simulink model "Vibro_Simulink Model"  (R2023a)
settings: Solver=VariableStepAuto  StartTime=0.0  StopTime=inf  RelTol=1e-3
undefined symbols (not defined in the file): f
libraries: instrumentlib x1
settings Model: Creator=Krishna Praveen  LastModifiedBy=Krishna Praveen

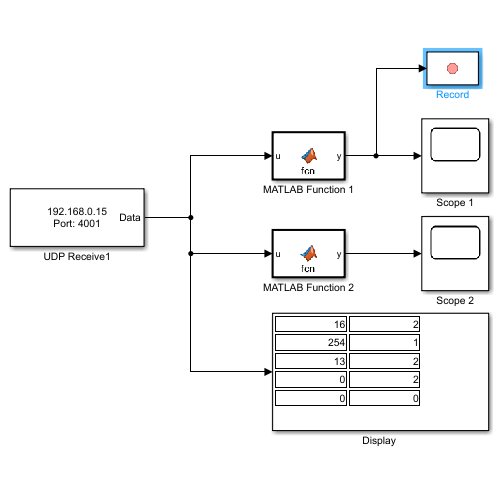
[thumbnail: Simulink's stored preview of the top-level diagram]
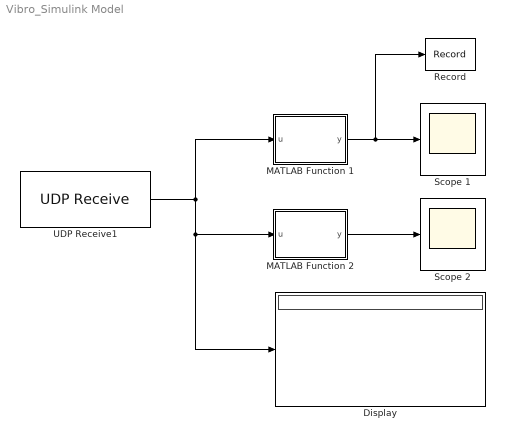
== system Vibro_Simulink Model ==
  "Display " : Display
  MATLAB Function 1 : MATLAB Function  TreatAsAtomicUnit=on
  MATLAB Function 2 : MATLAB Function  TreatAsAtomicUnit=on
  Record : Record  FileSettingsInternal="{\"entries\":[{\"content\":{\"excelSettings\":{\"content\":{},\"type\":\"Streamout.ExcelSettings\"}},\"type\":\"Streamout.FileSettingStorage\",\"uuid\":\"\"}],\"packageUris\":[\"http:\\/\\/schema.mathworks.com\\/mf0\\/streamout_blocks\\/R2020a\"],\"version\":\"1.0\"}"  SignalsInternal="{\"entries\":[{\"content\":{\"signals\":[{\"content\":{\"blockPath\":[],\"dimensions\":[1],\"domain\":\"\",\"lineColor\":\"#ff6929\",\"plots\":[1],\"port\":1,\"sid\":[\"\"],\"signalID\":128,\"signalName\":\"MATLAB Function 1\"},\"type\":\"RecordBlkView.Signal\",\"uuid\":\"\"}]},\"type\":\"RecordBlkView.InputSignals\",\"uuid\":\"\"}],\"packageUris\":[\"http:\\/\\/schema.mathworks.com\\/mf0\\/streamout_blocks\\/R2020a\"],\"version\":\"1.0\"}"  VisualizationBindings="{\"sparklinesplugin\":{\"info\":[{\"bindingParametersList\":[],\"subplotID\":1}]}}"
  Scope 1 : Scope
  Scope 2 : Scope
  UDP Receive1 : instrumentlib/UDP Receive  LocalAddress=192.168.0.15  LocalPort=4001  EnablePortSharing=off  Host=localhost  Port=9090  GetLatestData=off  DataSize=[ 1, 10 ]  DataType=uint8  ASCIIFormatting=%f,  Terminator=LF  CustomTerminator=10  ByteOrder=big-endian  EnableBlockingMode=on  Timeout=10  SampleTime=0.01  SimulateUsing=Interpreted execution
  wires:
  MATLAB Function 1/1(y) -> Record/1, Scope 1/1
  UDP Receive1/1 -> "Display "/1, MATLAB Function 2/1(u), MATLAB Function 1/1(u)
  MATLAB Function 2/1(y) -> Scope 2/1

== matlab function Vibro_Simulink Model/MATLAB Function 1 ==
  data: u input; y output
function y = fcn(u) 
%x = uint16(256*u(2) + u(1));
q = int16(u(2));
w = int16(u(1));
z = q * 256;
z = z + w;

a = int16(u(4));
b = int16(u(3));
c = a * 256;
c = c + b;

k = c - z;
y = k;

== matlab function Vibro_Simulink Model/MATLAB Function 2 ==
  data: u input; y output
function y = fcn(u) 
%x = uint16(256*u(6) + u(5));
q = int16(u(6));
w = int16(u(5));
z = q * 256;
z = z + w;

a = int16(u(8));
b = int16(u(7));
c = a * 256;
c = c + b;

k = c - z;
y = k;
